simulink model "EPD629_WilliamsJ_AS02_simulink"  (R2021b)
settings: Solver=VariableStepAuto  StartTime=0.0  StopTime=10.0  RelTol=1e-3
values from neighbouring files (symbols this model uses):
  AeroArea_m2 = 10    [EPD629_WilliamsJ_AS02.m]
  AeroDragCoef = 0.6    [EPD629_WilliamsJ_AS02.m]
  AirGasConstant_kJpkgK = 0.278    [EPD629_WilliamsJ_AS02.m]
  AmbientPress_kPa = 100    [EPD629_WilliamsJ_AS02.m]
  AmbientTemp_C = 20    [EPD629_WilliamsJ_AS02.m]
  CelsiusToKelvinConstant = 273.15    [EPD629_WilliamsJ_AS02.m]
  GravitationalAccel_mps2 = 9.8067    [EPD629_WilliamsJ_AS02.m]
  PitchAngleData_deg = [2 2]    [EPD629_WilliamsJ_AS02.m]
  PitchAnglePositionBP_m = [0 1e6]    [EPD629_WilliamsJ_AS02.m]
  RollingDragCoef = 0.005    [EPD629_WilliamsJ_AS02.m]
  VehicleMass_kg = 30000    [EPD629_WilliamsJ_AS02.m]
settings Model: Creator=jwilli42  LastModifiedBy=jwilli42

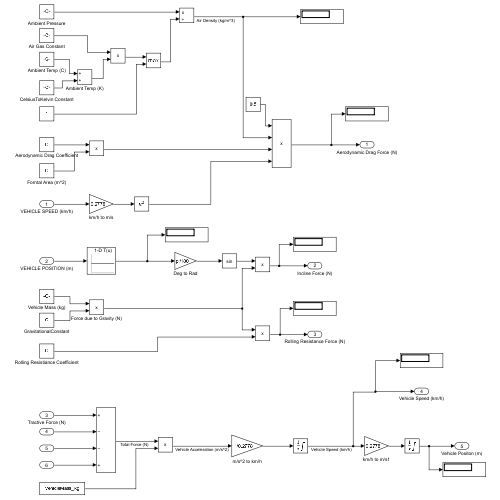
[thumbnail: Simulink's stored preview of the top-level diagram]
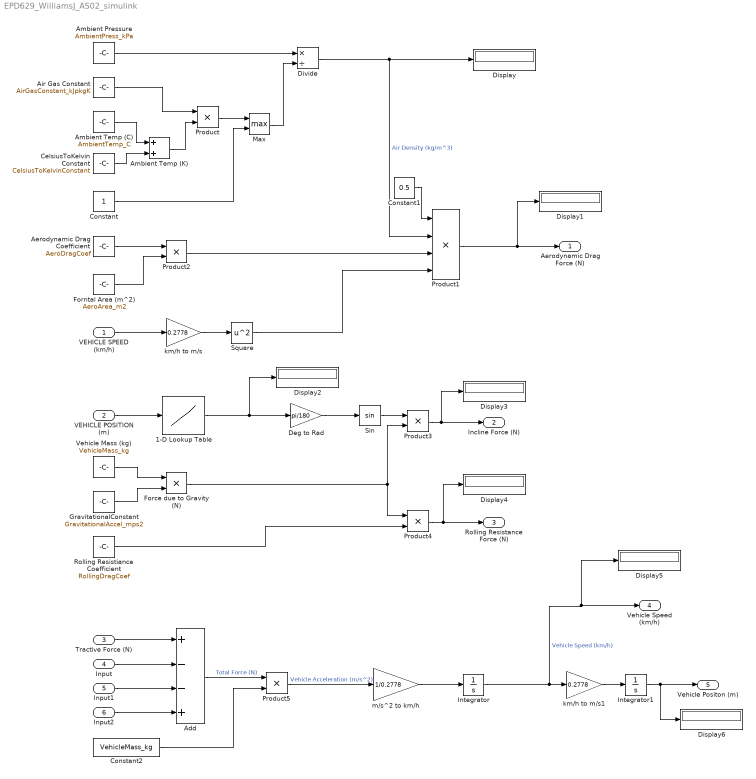
== system EPD629_WilliamsJ_AS02_simulink ==
  VEHICLE SPEED (km/h) : Inport
  VEHICLE POSITION (m) : Inport  Port=2
  Tractive Force (N) : Inport  Port=3
  Input : Inport  Port=4  OutputFunctionCall=on
  Input1 : Inport  Port=5
  Input2 : Inport  Port=6
  1-D Lookup Table : Lookup_n-D  NumberOfTableDimensions=1  BreakpointsForDimension1=PitchAnglePositionBP_m  Table=PitchAngleData_deg  ExtrapMethod=Clip  UseLastTableValue=on  InternalRulePriority=Speed  RndMeth=Simplest  InputSameDT=on
  Add : Sum  Inputs=+--+
  Aerodynamic Drag Coefficient : Constant  Value=AeroDragCoef
  Air Gas Constant : Constant  Value=AirGasConstant_kJpkgK
  Ambient Pressure : Constant  Value=AmbientPress_kPa
  Ambient Temp (C) : Constant  Value=AmbientTemp_C
  Ambient Temp (K) : Sum
  CelsiusToKelvin Constant : Constant  Value=CelsiusToKelvinConstant
  Constant : Constant
  Constant1 : Constant  Value=0.5
  Constant2 : Constant  Value=VehicleMass_kg
  Deg to Rad : Gain  Gain=pi/180
  Display{,1..6} (7 alike) : Display
  Divide : Product  Inputs=*/
  Force due to Gravity (N) : Product
  Forntal Area (m^2) : Constant  Value=AeroArea_m2
  GravitationalConstant : Constant  Value=GravitationalAccel_mps2
  Integrator : Integrator  LimitOutput=on  UpperSaturationLimit=150  LowerSaturationLimit=0
  Integrator1 : Integrator  LimitOutput=on  UpperSaturationLimit=1e6  LowerSaturationLimit=0
  Max : MinMax  Function=max  Inputs=2
  Product{,2..5} (5 alike) : Product
  Product1 : Product  Inputs=4
  Rolling Resistiance Coefficient : Constant  Value=RollingDragCoef
  Sin : Trigonometry
  Square : Math  Operator=square  SaturateOnIntegerOverflow=on
  Vehicle Mass (kg) : Constant  Value=VehicleMass_kg
  km/h to m/s : Gain  Gain=0.2778
  km/h to m/s1 : Gain  Gain=0.2778
  m/s^2 to km/h : Gain  Gain=1/0.2778
  Aerodynamic Drag Force (N) : Outport
  Incline Force (N) : Outport  Port=2
  Rolling Resistance Force (N) : Outport  Port=3
  Vehicle Speed (km/h) : Outport  Port=4
  Vehicle Positon (m) : Outport  Port=5
  wires:
  Ambient Temp (C)/1 -> Ambient Temp (K)/1
  CelsiusToKelvin Constant/1 -> Ambient Temp (K)/2
  Ambient Temp (K)/1 -> Product/2
  Air Gas Constant/1 -> Product/1
  Constant/1 -> Max/2
  Product/1 -> Max/1
  Max/1 -> Divide/2
  Ambient Pressure/1 -> Divide/1
  Divide/1 -> Display/1, Product1/2  "Air Density (kg/m^3)"
  Product1/1 -> Display1/1, Aerodynamic Drag Force (N)/1
  Aerodynamic Drag Coefficient/1 -> Product2/1
  Forntal Area (m^2)/1 -> Product2/2
  Product2/1 -> Product1/3
  Constant1/1 -> Product1/1
  Square/1 -> Product1/4
  VEHICLE SPEED (km/h)/1 -> km/h to m/s/1
  km/h to m/s/1 -> Square/1
  1-D Lookup Table/1 -> Display2/1, Deg to Rad/1
  Deg to Rad/1 -> Sin/1
  Sin/1 -> Product3/1
  Vehicle Mass (kg)/1 -> Force due to Gravity (N)/1
  GravitationalConstant/1 -> Force due to Gravity (N)/2
  Force due to Gravity (N)/1 -> Product4/1, Product3/2
  Rolling Resistiance Coefficient/1 -> Product4/2
  Product4/1 -> Display4/1, Rolling Resistance Force (N)/1
  Product3/1 -> Display3/1, Incline Force (N)/1
  VEHICLE POSITION (m)/1 -> 1-D Lookup Table/1
  Tractive Force (N)/1 -> Add/1
  Input/1 -> Add/2
  Input1/1 -> Add/3
  Input2/1 -> Add/4
  Add/1 -> Product5/1  "Total Force (N)"
  Constant2/1 -> Product5/2
  Product5/1 -> m/s^2 to km/h/1  "Vehicle Acceleration (m/s^2)"
  m/s^2 to km/h/1 -> Integrator/1
  Integrator/1 -> Vehicle Speed (km/h)/1, Display5/1, km/h to m/s1/1  "Vehicle Speed (km/h)"
  km/h to m/s1/1 -> Integrator1/1
  Integrator1/1 -> Display6/1, Vehicle Positon (m)/1
